simulink model "non_linear_PA"  (Simulink 7.4)
settings: Solver=VariableStepDiscrete  StartTime=0.0  StopTime=inf  RelTol=1e-3
undefined symbols (not defined in the file): dBm, Fs, Hz, One, rab_favorites, sided, Subsystem1, Two
libraries: dspsnks4 x2, dsparch4 x1, dspsrcs4 x1, commrflib2 x1, simulink x1, commfilt2 x1, commrandsrc2 x1, commdigbbndam3 x1
settings Model: Creator=dbenson  LastModifiedBy=Dick
settings DataIOCC: SignalLoggingName=sigsOut
settings OptimizationCC: BooleanDataType=off  InlineInvariantSignals=on  InitFltsAndDblsToZero=on
settings DebuggingCC: SaveWithParameterizedLinksMsg=none  SignalResolutionControl=TryResolveAllWithWarning  SolverPrmCheckMsg=none  MultiTaskDSMMsg=warning  MultiTaskCondExecSysMsg=none  StrictBusMsg=None
settings HardwareCC: TargetUnknown=on
settings RTWCC: IncludeERTFirstTime=on
settings GRTTargetCC: TargetFcnLib=ansi_tfl_tmw.mat

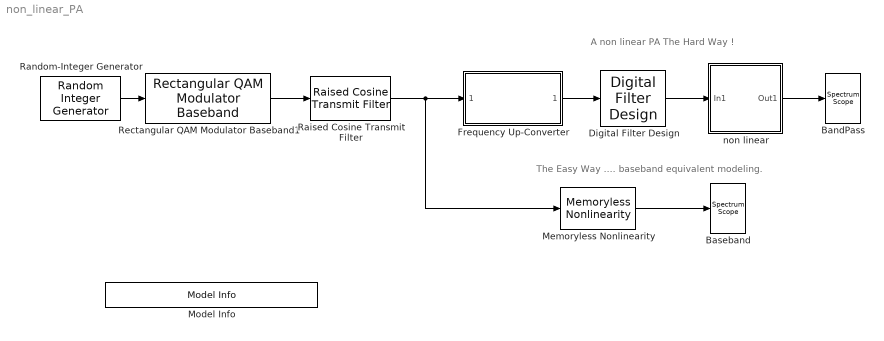
== system non_linear_PA ==
  note: A non linear PA The Hard Way !
  note: The Easy Way .... baseband equivalent modeling.
  BandPass : dspsnks4/Spectrum Scope  DialogController=dspdialog.SpectrumScope  DialogControllerArgs=DataTag0  SystemSampleTime=-1  ScopeProperties=on  Domain=Frequency  HorizSpan=1  UseBuffer=on  BufferSize=2048  Overlap=0  inpFftLenInherit=off  FFTlength=128  numAvg=20  DisplayProperties=off  AxisGrid=on  Memory=off  FrameNumber=on  AxisLegend=off  AxisZoom=off  OpenScopeAtSimStart=on  OpenScopeImmediately=off  FigPos=[121 342 425 265]  AxisProperties=off  XUnits=Hertz  XRange=One-sided ([0...Fs/2])  XDisplay=0  InheritXIncr=on  XIncr=1.0  XLabel=Samples  XLimit=Auto  YUnits=dBm/Hertz  XMax=1  XMin=0  YLabel=dBm/Hz  LineProperties=off  wintypeSpecScope=Hann  RsSpecScope=50  betaSpecScope=5  winsampSpecScope=Periodic  XAxisParamsVer=6.8
      settings: YMin=-140  YMax=-40
  Baseband : dspsnks4/Spectrum Scope  DialogController=dspdialog.SpectrumScope  DialogControllerArgs=DataTag1  SystemSampleTime=-1  ScopeProperties=on  Domain=Frequency  HorizSpan=1  UseBuffer=on  BufferSize=512  Overlap=0  inpFftLenInherit=off  FFTlength=128  numAvg=20  DisplayProperties=off  AxisGrid=on  Memory=off  FrameNumber=on  AxisLegend=off  AxisZoom=off  OpenScopeAtSimStart=on  OpenScopeImmediately=off  FigPos=[553 350 389 258]  AxisProperties=off  XUnits=Hertz  XRange=Two-sided ((-Fs/2...Fs/2])  XDisplay=0  InheritXIncr=on  XIncr=1.0  XLabel=Samples  XLimit=Auto  YUnits=dBm/Hertz  XMax=1  XMin=0  YLabel=dBm/Hz  LineProperties=off  wintypeSpecScope=Hann  RsSpecScope=50  betaSpecScope=5  winsampSpecScope=Periodic  XAxisParamsVer=6.8
      settings: YMin=-140  YMax=-40
  Digital Filter Design : dsparch4/Digital Filter Design  SystemSampleTime=-1  mwdsp_browser_bugfix_var=off
  Frequency Up-Converter : Subsystem  AncestorBlock=commblksprivate/Frequency Up-Converter  mask(Frequency Up-Converter){Fc=400*1e6, Ph=0, Tin=1/(8*40*1e6), Tout=1/(1600*1e6)}
      mask prompts: Fc "Carrier frequency (Hz):"; Ph "Carrier phase (rad):"; Tin "Input sample time:"; Tout "Output sample time:"
      mask help:
      | The Frequency Up-Converter translates the frequency of the baseband input signal to the carrier frequency.
      |
      | The input signal must be a sample-based scalar.
      mask init:
      | if (Tout>=1/(2*(Fc+1/Tin))) error('The reciprocal of the output sample time must be greater than twice the sum of the carrier frequency and the reciprocal of the input sample time.'); end;
      | 
      | if (Tin <= 1/Fc) error('The reciprocal of the input sample time must be less than the carrier frequency.'); end;
      | 
      | if (Tin<=Tout) error('The input sample time must be greater than the output sample time.'); end;
      mask Display: disp('Frequency\nUp-Converter');
  Memoryless Nonlinearity : commrflib2/Memoryless Nonlinearity  SystemSampleTime=-1  model_select=Hyperbolic tangent  linGaindB=0  GindB=0  iip3=20  am2pm=0  LPwrLimAMPM=10  UPwrLimAMPM=inf  amam=[2.1587 1.1517]  ampm=[4.0033 9.1040]  x=[8.1081 1.5413 6.5202 -0.0718]  y=[4.6645 2.0965 10.88 -0.003]  p=0.5  GoutdB=0  vsat=1
  Model Info : simulink/Model-Wide Utilities/Model Info  SystemSampleTime=-1  InitialBlockCM=None  BlockCM=None  Frame=on  DisplayStringWithTags=Copywrite 2005-2010 The MathWorks, Inc.  HorizontalTextAlignment=Center  LeftAlignmentValue=0.5  SourceBlockDiagram=non_linear_PA  TagMaxNumber=20
  Raised Cosine Transmit Filter : commfilt2/Raised Cosine Transmit Filter  DialogController=dspDDGCreate  DialogControllerArgs=DataTag3  SystemSampleTime=-1  filtType=Square root  D=8  R=0.1  sampMode=Mute  saveAsFlag=0  framing=Maintain input frame size  N=8  checkGain=Normalized  filterGain=1  checkCoeff=off  variableName=rcTxFilt  launchFVT=off  roundingMode=Floor  overflowMode=off
  Random-Integer Generator : commrandsrc2/Random Integer Generator  SystemSampleTime=-1  mul=4  seed=[12345]  Ts=1/(40*1e6)  frameBased=off  sampPerFrame=1  orient=off  outDataType=double
  Rectangular QAM Modulator Baseband1 : commdigbbndam3/Rectangular QAM Modulator Baseband  DialogController=commDDGCreate  DialogControllerArgs=DataTag4  M=4  InType=Integer  Enc=Binary  Mapping=[0:15]  PowType=Peak Power  MinDist=2  AvgPow=1  PeakPow=1  Ph=0  outDtype=double  outWordLen=16  outUDDataType=sfix(16)  outFracLenMode=Best precision  outFracLen=15
  non linear : Subsystem  AncestorBlock=rab_favorites/Subsystem1  mask{alpha=.2}
      mask init:
      | x=-3:0.01:3;  y= (1/alpha)*tanh(alpha*x) ;
      mask Display: plot(x,y)
  wires:
  Rectangular QAM Modulator Baseband1/1 -> Raised Cosine Transmit Filter/1
  Frequency Up-Converter/1("  ") -> Digital Filter Design/1
  Digital Filter Design/1 -> non linear/1(In1)
  non linear/1(Out1) -> BandPass/1
  Random-Integer Generator/1 -> Rectangular QAM Modulator Baseband1/1
  Memoryless Nonlinearity/1 -> Baseband/1
  Raised Cosine Transmit Filter/1 -> Frequency Up-Converter/1(" "), Memoryless Nonlinearity/1

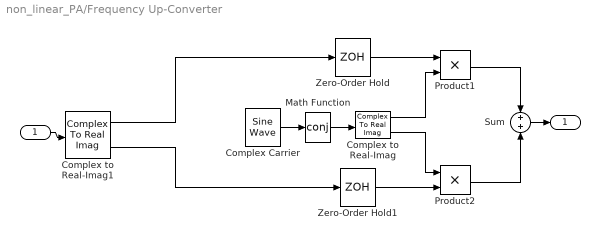
== system non_linear_PA/Frequency Up-Converter ==
  " " : Inport  OutDataType=sfix(16)  OutScaling=2^0
  Complex Carrier : dspsrcs4/Sine Wave  Amplitude=sqrt(2)  Frequency=Fc  Phase=Ph  SampleMode=Discrete  OutComplex=Complex  CompMethod=Trigonometric fcn  TableSize=Speed  SampleTime=Tout  SamplesPerFrame=1  dataType=double  wordLen=16  udDataType=sfix(16)  fracBitsMode=Best precision  numFracBits=14  ResetState=Restart at time zero
  Complex to Real-Imag : ComplexToRealImag
  Complex to Real-Imag1 : ComplexToRealImag
  Math Function : Math  Operator=conj  OutDataType=sfix(16)  OutScaling=2^0  SaturateOnIntegerOverflow=on
  Product1 : Product  OutDataType=sfix(16)  OutScaling=2^0  SaturateOnIntegerOverflow=on  InputSameDT=on  OutDataTypeStr=Inherit: Same as first input
  Product2 : Product  OutDataType=sfix(16)  OutScaling=2^0  SaturateOnIntegerOverflow=on  InputSameDT=on  OutDataTypeStr=Inherit: Same as first input
  Sum : Sum  Inputs=+|+  OutDataType=sfix(16)  OutScaling=2^0  SaturateOnIntegerOverflow=on  InputSameDT=on  OutDataTypeStr=Inherit: Same as first input
  Zero-Order Hold : ZeroOrderHold  SampleTime=Tout
  Zero-Order Hold1 : ZeroOrderHold  SampleTime=Tout
  "  " : Outport  OutDataType=sfix(16)  OutScaling=2^0
  wires:
  Zero-Order Hold1/1 -> Product2/2
  Zero-Order Hold/1 -> Product1/1
  Complex Carrier/1 -> Math Function/1
  Math Function/1 -> Complex to Real-Imag/1
  " "/1 -> Complex to Real-Imag1/1
  Complex to Real-Imag1/2 -> Zero-Order Hold1/1
  Complex to Real-Imag1/1 -> Zero-Order Hold/1
  Complex to Real-Imag/1 -> Product1/2
  Complex to Real-Imag/2 -> Product2/1
  Product1/1 -> Sum/1
  Product2/1 -> Sum/2
  Sum/1 -> "  "/1

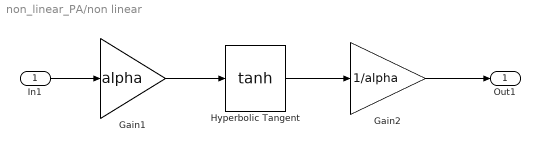
== system non_linear_PA/non linear ==
  In1 : Inport  OutDataType=sfix(16)  OutScaling=2^0
  Gain1 : Gain  Gain=alpha  ParameterDataType=sfix(16)  ParameterScaling=2^0  OutDataType=sfix(16)  OutScaling=2^0  SaturateOnIntegerOverflow=on  OutDataTypeStr=Inherit: Same as input  ParamDataTypeStr=Inherit: Same as input
  Gain2 : Gain  Gain=1/alpha  ParameterDataType=sfix(16)  ParameterScaling=2^0  OutDataType=sfix(16)  OutScaling=2^0  SaturateOnIntegerOverflow=on  OutDataTypeStr=Inherit: Same as input  ParamDataTypeStr=Inherit: Same as input
  Hyperbolic Tangent : Trigonometry  Operator=tanh
  Out1 : Outport  OutDataType=sfix(16)  OutScaling=2^0
  wires:
  Hyperbolic Tangent/1 -> Gain2/1
  In1/1 -> Gain1/1
  Gain2/1 -> Out1/1
  Gain1/1 -> Hyperbolic Tangent/1
